simulink model "single_generator_initFinish"  (R2014a)
settings: Solver=ode23tb  StartTime=0.0  StopTime=10.0  MaxStep=1e-3  RelTol=1e-4
libraries: powerlib x4
settings Model: Creator=scastro  LastModifiedBy=cosorio
settings DebuggingCC: UnderspecifiedInitializationDetection=Classic  MultiTaskDSMMsg=warning  MultiTaskCondExecSysMsg=none
settings RTWCC: IncludeERTFirstTime=on

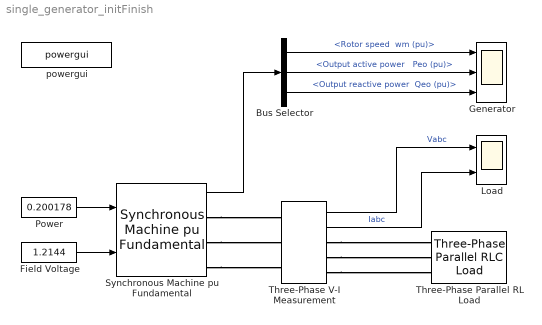
== system single_generator_initFinish ==
  Bus Selector : BusSelector  OutputSignals="Mechanical.Rotor speed  wm (pu),Output active power   Peo (pu),Output reactive power  Qeo (pu)"
  Field Voltage : Constant  Value=1.2144
  Generator : Scope  NumInputPorts=3
      settings: YMin=0~0~0  YMax=2~1~1
  Load : Scope  NumInputPorts=2
      settings: YMin=-20000~-5000  YMax=20000~5000
  Power : Constant  Value=0.200178
  Synchronous Machine pu Fundamental : powerlib/Machines/Synchronous Machine pu Fundamental  PresetModel=No  MechanicalLoad=Mechanical power Pm  ShowDetailedParameters=on  RotorType=Salient-pole  Units=per unit fundamental parameters  MeasurementBus=off  NominalParameters="[ 100e6  13800   60]"  Stator="[ 2.85E-03  0.114  1.19  0.36 ]"  Field="[ 5.79E-04  0.114]"  Dampers2=[0.0652, 0.5134, 0.0287, 0.2553, 7.765e-3, 0.9167 ]  Dampers1="[ 1.17E-02  0.182  1.97E-02  0.384 ]"  Mechanical=[ 3.7 0 2]  PolePairs=2  InitialConditions=[0 -84.9674 0.25 0.25 0.25 -36.8699 -156.87 83.1301 1.2144]  SetSaturation=off  Saturation=[0.6404,0.7127,0.8441,0.9214,0.9956,1.082,1.19,1.316,1.457;0.7,0.7698,0.8872,0.9466,0.9969,1.046,1.1,1.151,1.201]  LoadFlowParameters=[2 20000 0 0 0]  TsPowergui=0  TsBlock=-1  IterativeModel=Trapezoidal non iterative  BusType=PQ  Pref=0  Qref=0  Qmin=-inf  Qmax=inf  PLF=0  QLF=0
      settings: AttributesFormatString=%<NominalParameters>
  Three-Phase Parallel RL Load : powerlib/Elements/Three-Phase Parallel RLC Load  LConnTagsString=A|B|C  Configuration=Y (grounded)  NominalVoltage=13800  NominalFrequency=60  ActivePower=20e6  InductivePower=15e6  CapacitivePower=0  Measurements=None  LoadType=constant Z
      settings: AttributesFormatString=|
      | Vn = %<NominalVoltage> Vrms
      | f = %<NominalFrequency> Hz
      | P = %<ActivePower> W
      | Q = %<InductivePower> Var
  Three-Phase V-I Measurement : powerlib/Measurements/Three-Phase V-I Measurement  VoltageMeasurement=phase-to-ground  SetLabelV=off  LabelV=Vabc  Vpu=off  VpuLL=off  CurrentMeasurement=yes  SetLabelI=off  LabelI=Iabc  Ipu=off  Pbase=100e6  Vbase=500e3  OutputType=Complex  PhasorSimulation=off  PSBequivalent=0
  powergui : powerlib/powergui  Priority=1  SimulationMode=Continuous  SolverType=Tustin  SampleTime=50e-6  frequency=60  SPID=off  DisableSnubberDevices=off  DisableRonSwitches=off  DisableVfSwitches=off  SwTol=0  Interpol=off  DisplayEquations=off  Ts=0  methode=off  frequencyindice=60  Pbase=100e6  ErrMax=1e-4  Iterations=50  UnitsV=kV  UnitsW=MW  FunctionMessages=off  echomessages=off  HookPort=off  EnableUseOfTLC=off  x0status=blocks  RestoreLinks=warning  ResistiveCurrentMeasurement=off  Frange=[0:2:500]  Ylog=off  Xlog=on  ShowGrid=off  save=off  variable=ZData  structure=0  ZoomFFT=off  StartTime=0.0  cycles=1  DisplayStyle=1  fundamental=60  FreqAxis=off  MaxFrequency=1000  frequencyindicesteady=1  RmsSteady=1  display=off
  wires:
  Three-Phase V-I Measurement/2 -> Load/2  "Iabc"
  Three-Phase V-I Measurement/1 -> Load/1  "Vabc"
  Power/1 -> Synchronous Machine pu Fundamental/1
  Field Voltage/1 -> Synchronous Machine pu Fundamental/2
  Synchronous Machine pu Fundamental/1 -> Bus Selector/1
  Bus Selector/3 -> Generator/3  "<Output reactive power  Qeo (pu)>"
  Bus Selector/2 -> Generator/2  "<Output active power   Peo (pu)>"
  Bus Selector/1 -> Generator/1  "<Rotor speed  wm (pu)>"
  connections:
  Synchronous Machine pu Fundamental/RConn1 -- Three-Phase V-I Measurement/LConn1
  Synchronous Machine pu Fundamental/RConn2 -- Three-Phase V-I Measurement/LConn2
  Synchronous Machine pu Fundamental/RConn3 -- Three-Phase V-I Measurement/LConn3
  Three-Phase V-I Measurement/RConn1 -- Three-Phase Parallel RL Load/LConn1
  Three-Phase V-I Measurement/RConn2 -- Three-Phase Parallel RL Load/LConn2
  Three-Phase V-I Measurement/RConn3 -- Three-Phase Parallel RL Load/LConn3
